simulink model "Main2016a"  (R2016a)
settings: Solver=ode45  StartTime=0.0  StopTime=t_end  FixedStep=st  MaxStep=st  RelTol=1e-3
values from neighbouring files (symbols this model uses):
  A = eye(16,16)    [full_input_list.m]
  counter = 0    [full_input_list.m]
  I_1 = [m*(zl^2+xyl^2)/12 0 0 ;          0 m*(zl^2+xyl^2)/12 0 ;          0 0 m*(2*xyl^2)/12 ] + 1e-6*(rand(3)-0.5)    [initACS.m]
  I_1_inv = inv(I_1)    [initACS.m]
  I_2 = [m*(zl^2+xyl^2)/12 0 0 ;          0 m*(zl^2+xyl^2)/12 0 ;          0 0 m*(2*xyl^2)/12 ] + 1e-6*(rand(3)-0.5)    [initACS.m]
  I_2_inv = inv(I_2)    [initACS.m]
  I_3 = [m*(zl^2+xyl^2)/12 0 0 ;          0 m*(zl^2+xyl^2)/12 0 ;          0 0 m*(2*xyl^2)/12 ] + 1e-6*(rand(3)-0.5)    [initACS.m]
  I_3_inv = inv(I_3)    [initACS.m]
  kd = 0.5    [full_input_list.m]    (also in initACS.m = 0.01)
  kp = 1    [full_input_list.m]    (also in initACS.m = 0.01)
  OpModes = [0 0 0]    [full_input_list.m]
  OpTimes = [0 1 2]    [full_input_list.m]
  SeperationTime = 30000    [full_input_list.m]
  state1_i = [ 0 0 0 , 0 0 0 , q4_0', w0_N]'    [full_input_list.m]
  state2_i = [ 0 0 (teth_length+side1Dim(1)/2+centerDim(3)/2+10*eps) , 0 -.1 0 ,      q4_0_Cube2' , w0_N ]'    [full_input_list.m]
  state3_i = [ 0 0 -(teth_length+side1Dim(1)/2+centerDim(3)/2+10*eps), 0 .1 0 ,      q4_0_Cube3' , w0_N ]'    [full_input_list.m]
  teth_k = teth_area*teth_modulus/teth_length    (= 33772.1210261)    [full_input_list.m]    (also in initACS.m = 10)
  teth_lo = 30    [full_input_list.m]    (also in initACS.m)
undefined symbols (not defined in the file or in its folder): DiscIntNeverNeededParam, Inertia, km, n, SolarDeployTime, solarpanel1_i, solarpanel2_i
libraries: SimMainLibrary x11, aerolibutil x10, simulink x1, vrlib x1, dspmathops x1
(part 1 of 2)
settings Model: Creator=dtk42  LastModifiedBy=cjtho
settings SolverCC: ZeroCrossAlgorithm=Adaptive
settings GRTTargetCC: GeneratePreprocessorConditionals=Use local settings

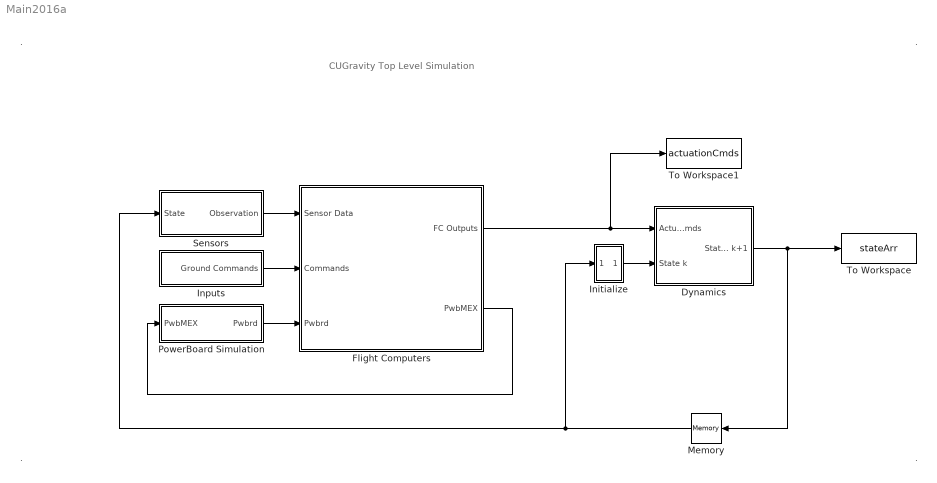
== system Main2016a ==
  note: .
  note: .
  note: .
  note: .
  note: CUGravity Top Level Simulation
  Dynamics : Subsystem
  Flight Computers : Subsystem
  Initialize : Subsystem
  Inputs : Subsystem
  Memory : Memory  InheritSampleTime=on
  PowerBoard Simulation : Subsystem
  Sensors : Subsystem
  To Workspace : ToWorkspace  VariableName=stateArr  SaveFormat=Timeseries  SampleTime=-1
  To Workspace1 : ToWorkspace  VariableName=actuationCmds  SaveFormat=Timeseries  SampleTime=-1
  wires:
  Sensors/1(Observation) -> Flight Computers/1(Sensor Data)
  Flight Computers/1(FC Outputs) -> Dynamics/1(Actuation Cmds), To Workspace1/1
  Initialize/1(xi) -> Dynamics/2(State k)
  Dynamics/1(State k+1) -> Memory/1, To Workspace/1
  Memory/1 -> Initialize/1(x), Sensors/1(State)
  Inputs/1(Ground Commands) -> Flight Computers/2(Commands)
  PowerBoard Simulation/1(Pwbrd) -> Flight Computers/3(Pwbrd)
  Flight Computers/2(PwbMEX) -> PowerBoard Simulation/1(PwbMEX)

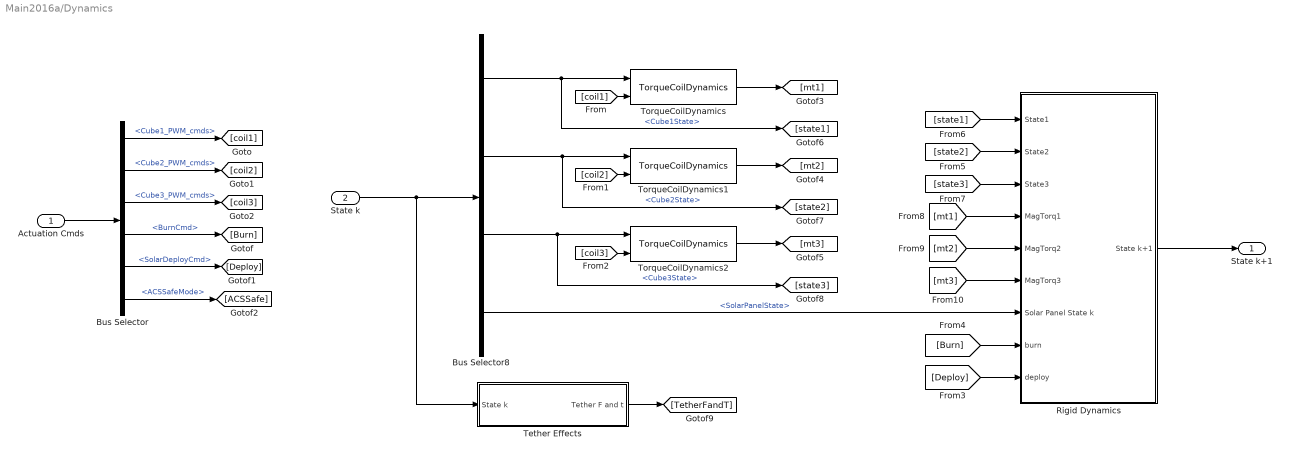
== system Main2016a/Dynamics ==
  Actuation Cmds : Inport
  State k : Inport  Port=2
  Bus Selector : BusSelector  OutputSignals=Cube1_PWM_cmds,Cube2_PWM_cmds,Cube3_PWM_cmds,BurnCmd,SolarDeployCmd,ACSSafeMode
  Bus Selector8 : BusSelector  OutputSignals=Cube1State,Cube2State,Cube3State,SolarPanelState
  Rigid Dynamics : Subsystem
  Tether Effects : Subsystem
  TorqueCoilDynamics : SimMainLibrary/TorqueCoilDynamics
  TorqueCoilDynamics1 : SimMainLibrary/TorqueCoilDynamics
  TorqueCoilDynamics2 : SimMainLibrary/TorqueCoilDynamics
  State k+1 : Outport
  wires:
  Bus Selector8/1 -> [state1], TorqueCoilDynamics/1  "<Cube1State>"
  Bus Selector8/2 -> TorqueCoilDynamics1/1, [state2]  "<Cube2State>"
  Bus Selector8/3 -> [state3], TorqueCoilDynamics2/1  "<Cube3State>"
  Bus Selector/1 -> [coil1]  "<Cube1_PWM_cmds>"
  Bus Selector/2 -> [coil2]  "<Cube2_PWM_cmds>"
  Bus Selector/3 -> [coil3]  "<Cube3_PWM_cmds>"
  [coil1] -> TorqueCoilDynamics/2
  [coil2] -> TorqueCoilDynamics1/2
  [coil3] -> TorqueCoilDynamics2/2
  Actuation Cmds/1 -> Bus Selector/1
  Bus Selector/4 -> [Burn]  "<BurnCmd>"
  Bus Selector/5 -> [Deploy]  "<SolarDeployCmd>"
  State k/1 -> Tether Effects/1(State k), Bus Selector8/1
  Rigid Dynamics/1(State k+1) -> State k+1/1
  Bus Selector/6 -> [ACSSafe]  "<ACSSafeMode>"
  TorqueCoilDynamics/1 -> [mt1]
  TorqueCoilDynamics1/1 -> [mt2]
  TorqueCoilDynamics2/1 -> [mt3]
  Tether Effects/1(Tether F and t) -> [TetherFandT]
  [Burn] -> Rigid Dynamics/8(burn)
  [Deploy] -> Rigid Dynamics/9(deploy)
  [state2] -> Rigid Dynamics/2(State2)
  [state1] -> Rigid Dynamics/1(State1)
  [state3] -> Rigid Dynamics/3(State3)
  [mt1] -> Rigid Dynamics/4(MagTorq1)
  [mt2] -> Rigid Dynamics/5(MagTorq2)
  [mt3] -> Rigid Dynamics/6(MagTorq3)
  Bus Selector8/4 -> Rigid Dynamics/7(Solar Panel State k)  "<SolarPanelState>"

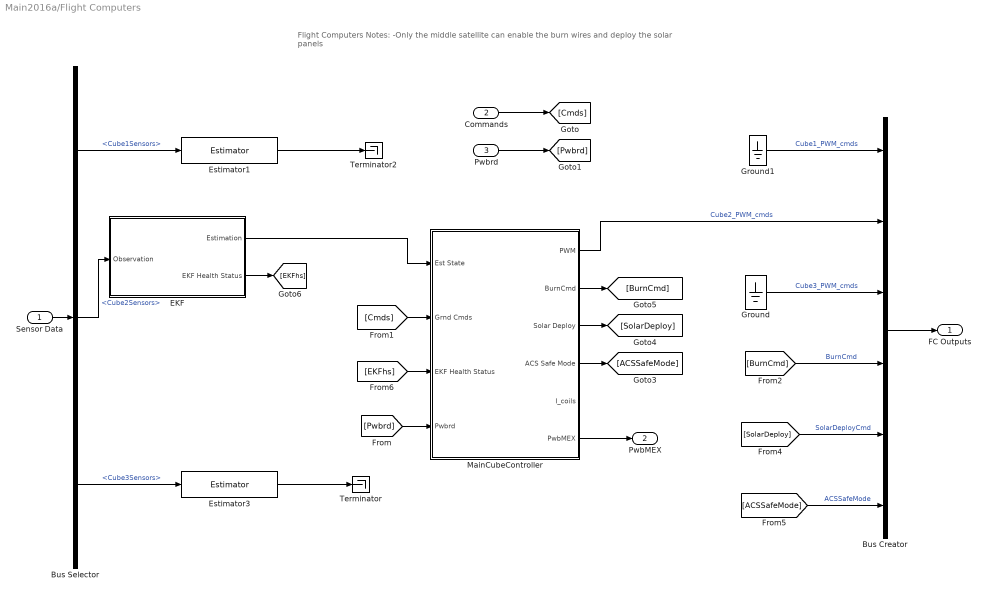
== system Main2016a/Flight Computers ==
  note: Flight Computers
      | Notes:
      | -Only the middle satellite can enable the burn wires and deploy the solar panels
  Sensor Data : Inport
  Commands : Inport  Port=2
  Pwbrd : Inport  Port=3
  Bus Creator : BusCreator  Inputs=6
  Bus Selector : BusSelector  OutputSignals=Cube1Sensors,Cube2Sensors,Cube3Sensors
  EKF : Subsystem  AncestorBlock=SimMainLibrary/Estimator
  Estimator1 : SimMainLibrary/Estimator
  Estimator3 : SimMainLibrary/Estimator
  Ground : Ground
  Ground1 : Ground
  MainCubeController : Subsystem  AncestorBlock=SimMainLibrary/MainCubeController
  Terminator : Terminator
  Terminator2 : Terminator
  FC Outputs : Outport
  PwbMEX : Outport  Port=2
  wires:
  Sensor Data/1 -> Bus Selector/1
  Bus Selector/1 -> Estimator1/1  "<Cube1Sensors>"
  EKF/1(Estimation) -> MainCubeController/1(Est State)
  Bus Selector/2 -> EKF/1(Observation)  "<Cube2Sensors>"
  MainCubeController/1(PWM) -> Bus Creator/2  "Cube2_PWM_cmds"
  Estimator3/1 -> Terminator/1
  Bus Selector/3 -> Estimator3/1  "<Cube3Sensors>"
  Estimator1/1 -> Terminator2/1
  Ground1/1 -> Bus Creator/1  "Cube1_PWM_cmds"
  Bus Creator/1 -> FC Outputs/1
  Ground/1 -> Bus Creator/3  "Cube3_PWM_cmds"
  Commands/1 -> [Cmds]
  [Cmds] -> MainCubeController/2(Grnd Cmds)
  MainCubeController/4(ACS Safe Mode) -> [ACSSafeMode]
  MainCubeController/3(Solar Deploy) -> [SolarDeploy]
  MainCubeController/2(BurnCmd) -> [BurnCmd]
  [BurnCmd] -> Bus Creator/4  "BurnCmd"
  [SolarDeploy] -> Bus Creator/5  "SolarDeployCmd"
  [ACSSafeMode] -> Bus Creator/6  "ACSSafeMode"
  EKF/2(EKF Health Status) -> [EKFhs]
  [EKFhs] -> MainCubeController/3("EKF Health Status ")
  Pwbrd/1 -> [Pwbrd]
  [Pwbrd] -> MainCubeController/4(Pwbrd)
  MainCubeController/6(PwbMEX) -> PwbMEX/1

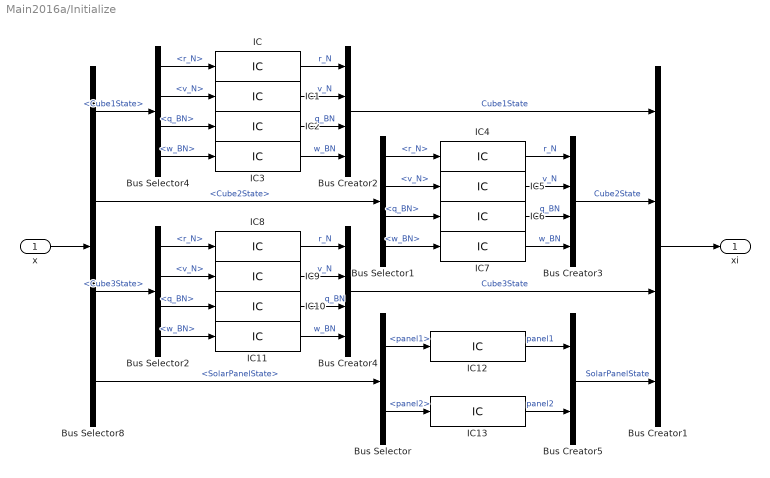
== system Main2016a/Initialize ==
  x : Inport
  Bus Creator1 : BusCreator  Inputs=4
  Bus Creator2 : BusCreator  Inputs='r_N','v_N','q_BN','w_BN'
  Bus Creator3 : BusCreator  Inputs='r_N','v_N','q_BN','w_BN'
  Bus Creator4 : BusCreator  Inputs='r_N','v_N','q_BN','w_BN'
  Bus Creator5 : BusCreator  Inputs='panel1','panel2'
  Bus Selector : BusSelector  OutputSignals=panel1,panel2
  Bus Selector1 : BusSelector  OutputSignals=r_N,v_N,q_BN,w_BN
  Bus Selector2 : BusSelector  OutputSignals=r_N,v_N,q_BN,w_BN
  Bus Selector4 : BusSelector  OutputSignals=r_N,v_N,q_BN,w_BN
  Bus Selector8 : BusSelector  OutputSignals=Cube1State,Cube2State,Cube3State,SolarPanelState
  IC : InitialCondition  Value=state1_i(1:3)
  IC1 : InitialCondition  Value=state1_i(4:6)
  IC10 : InitialCondition  Value=state3_i(7:10)
  IC11 : InitialCondition  Value=state3_i(11:13)
  IC12 : InitialCondition  Value=solarpanel1_i(1:4)
  IC13 : InitialCondition  Value=solarpanel2_i(1:4)
  IC2 : InitialCondition  Value=state1_i(7:10)
  IC3 : InitialCondition  Value=state1_i(11:13)
  IC4 : InitialCondition  Value=state2_i(1:3)
  IC5 : InitialCondition  Value=state2_i(4:6)
  IC6 : InitialCondition  Value=state2_i(7:10)
  IC7 : InitialCondition  Value=state2_i(11:13)
  IC8 : InitialCondition  Value=state3_i(1:3)
  IC9 : InitialCondition  Value=state3_i(4:6)
  xi : Outport
  wires:
  Bus Selector4/3 -> IC2/1  "<q_BN>"
  x/1 -> Bus Selector8/1
  Bus Creator1/1 -> xi/1
  Bus Selector8/1 -> Bus Selector4/1  "<Cube1State>"
  Bus Selector4/4 -> IC3/1  "<w_BN>"
  Bus Selector4/1 -> IC/1  "<r_N>"
  Bus Creator2/1 -> Bus Creator1/1  "Cube1State"
  Bus Selector4/2 -> IC1/1  "<v_N>"
  IC/1 -> Bus Creator2/1  "r_N"
  IC1/1 -> Bus Creator2/2  "v_N"
  IC2/1 -> Bus Creator2/3  "q_BN"
  IC3/1 -> Bus Creator2/4  "w_BN"
  Bus Selector1/3 -> IC6/1  "<q_BN>"
  Bus Selector1/4 -> IC7/1  "<w_BN>"
  Bus Selector1/1 -> IC4/1  "<r_N>"
  Bus Selector1/2 -> IC5/1  "<v_N>"
  Bus Selector8/2 -> Bus Selector1/1  "<Cube2State>"
  Bus Selector2/3 -> IC10/1  "<q_BN>"
  Bus Selector2/4 -> IC11/1  "<w_BN>"
  Bus Selector2/1 -> IC8/1  "<r_N>"
  Bus Selector2/2 -> IC9/1  "<v_N>"
  Bus Selector8/3 -> Bus Selector2/1  "<Cube3State>"
  IC4/1 -> Bus Creator3/1  "r_N"
  IC5/1 -> Bus Creator3/2  "v_N"
  IC6/1 -> Bus Creator3/3  "q_BN"
  IC7/1 -> Bus Creator3/4  "w_BN"
  Bus Creator4/1 -> Bus Creator1/3  "Cube3State"
  IC8/1 -> Bus Creator4/1  "r_N"
  IC9/1 -> Bus Creator4/2  "v_N"
  IC10/1 -> Bus Creator4/3  "q_BN"
  IC11/1 -> Bus Creator4/4  "w_BN"
  Bus Creator3/1 -> Bus Creator1/2  "Cube2State"
  Bus Selector8/4 -> Bus Selector/1  "<SolarPanelState>"
  Bus Creator5/1 -> Bus Creator1/4  "SolarPanelState"
  IC12/1 -> Bus Creator5/1  "panel1"
  IC13/1 -> Bus Creator5/2  "panel2"
  Bus Selector/1 -> IC12/1  "<panel1>"
  Bus Selector/2 -> IC13/1  "<panel2>"

== system Main2016a/Inputs ==
  Bus Creator : BusCreator  Inputs=3
  Choose Mode : MATLAB Function  TreatAsAtomicUnit=on
      settings: PermitHierarchicalResolution=ParametersOnly
  Clock : Clock
  Constant : Constant  Value=OpModes
  Constant1 : Constant  Value=OpTimes
  Constant2 : Constant  Value=SeperationTime
  Constant3 : Constant  Value=SolarDeployTime
  Ground Commands : Outport
  wires:
  Constant/1 -> Choose Mode/3(OpModes)
  Constant1/1 -> Choose Mode/2(OpTimes)
  Clock/1 -> Choose Mode/1(time)
  Constant2/1 -> Choose Mode/4(SeperationTime)
  Choose Mode/1(OM) -> Bus Creator/1  "OpMode"
  Choose Mode/2(SEPC) -> Bus Creator/2  "SeperationCommand"
  Bus Creator/1 -> Ground Commands/1
  Constant3/1 -> Choose Mode/5(SolarDeployTime)
  Choose Mode/3(SDC) -> Bus Creator/3  "SolarDeployCommand"

== system Main2016a/PowerBoard Simulation ==
  PwbMEX : Inport
  Bus Creator : BusCreator  Inputs=2
  Bus Creator1 : BusCreator  Inputs=8
  Bus Creator2 : BusCreator  Inputs=3
  Bus Creator3 : BusCreator  Inputs=2
  Bus Creator4 : BusCreator  Inputs=2
  Choose Mode : MATLAB Function  TreatAsAtomicUnit=on
      settings: PermitHierarchicalResolution=ParametersOnly
  Clock : Clock
  Constant : Constant  Value=OpModes
  Constant1 : Constant  Value=OpTimes
  Constant2 : Constant  Value=SeperationTime
  Constant3 : Constant  Value=SolarDeployTime
  Sensor Ak Signals : Subsystem
  Terminator : Terminator
  Torquer Shunts : Subsystem
  Pwbrd : Outport
  wires:
  Constant/1 -> Choose Mode/4(OpModes)
  Constant1/1 -> Choose Mode/3(OpTimes)
  Clock/1 -> Choose Mode/2(time)
  Constant2/1 -> Choose Mode/5(SeperationTime)
  Choose Mode/1(OM) -> Bus Creator/1  "PbOpMode"
  Choose Mode/2(SEPC) -> Bus Creator/2  "PbSepCmmd"
  Bus Creator/1 -> Bus Creator4/1  "PwbrdCmmds"
  Constant3/1 -> Choose Mode/6(SolarDeployTime)
  Choose Mode/3(SDC) -> Terminator/1  "SolarDeployCommand"
  Sensor Ak Signals/4(Out4) -> Bus Creator1/4  "Accel2Ak"
  Sensor Ak Signals/3(Out3) -> Bus Creator1/3  "Accel1Ak"
  Sensor Ak Signals/1(Out1) -> Bus Creator1/1  "Mag1Ak"
  Sensor Ak Signals/2(Out2) -> Bus Creator1/2  "Mag2Ak"
  Bus Creator1/1 -> Bus Creator3/1  "SensorsAk"
  Torquer Shunts/1(Torquer X1 Shunt) -> Bus Creator2/1  "TC_X1"
  Torquer Shunts/2(Torquer Y1 Shunt) -> Bus Creator2/2  "TC_Y1"
  Torquer Shunts/3(Torquer Z1 Shunt) -> Bus Creator2/3  "TC_Z1"
  Bus Creator2/1 -> Bus Creator3/2  "TorquerAk"
  Bus Creator3/1 -> Bus Creator4/2  "ADCSAks"
  Bus Creator4/1 -> Pwbrd/1
  Sensor Ak Signals/5(Out5) -> Bus Creator1/5  "Gyro1Ak"
  Sensor Ak Signals/6(Out6) -> Bus Creator1/6  "Gyro2Ak"
  Sensor Ak Signals/7(Out7) -> Bus Creator1/7  "SunS1Ak"
  Sensor Ak Signals/8(Out8) -> Bus Creator1/8  "SunS2Ak"
  PwbMEX/1 -> Choose Mode/1(PwbMEX)

== system Main2016a/Sensors ==
  State : Inport
  Bus Creator1 : BusCreator  Inputs=3
  Bus Selector1 : BusSelector  OutputSignals=Cube1State,Cube2State,Cube3State
  Rate Transition : RateTransition
  SensorsBlock1 : SimMainLibrary/SensorsBlock
  SensorsBlock2 : SimMainLibrary/SensorsBlock
  SensorsBlock3 : SimMainLibrary/SensorsBlock
  Observation : Outport
  wires:
  Bus Creator1/1 -> Observation/1
  State/1 -> Rate Transition/1
  Bus Selector1/1 -> SensorsBlock3/1  "<Cube1State>"
  SensorsBlock3/1 -> Bus Creator1/1  "Cube1Sensors"
  SensorsBlock2/1 -> Bus Creator1/3  "Cube3Sensors"
  SensorsBlock1/1 -> Bus Creator1/2  "Cube2Sensors"
  Bus Selector1/2 -> SensorsBlock1/1  "<Cube2State>"
  Bus Selector1/3 -> SensorsBlock2/1  "<Cube3State>"
  Rate Transition/1 -> Bus Selector1/1

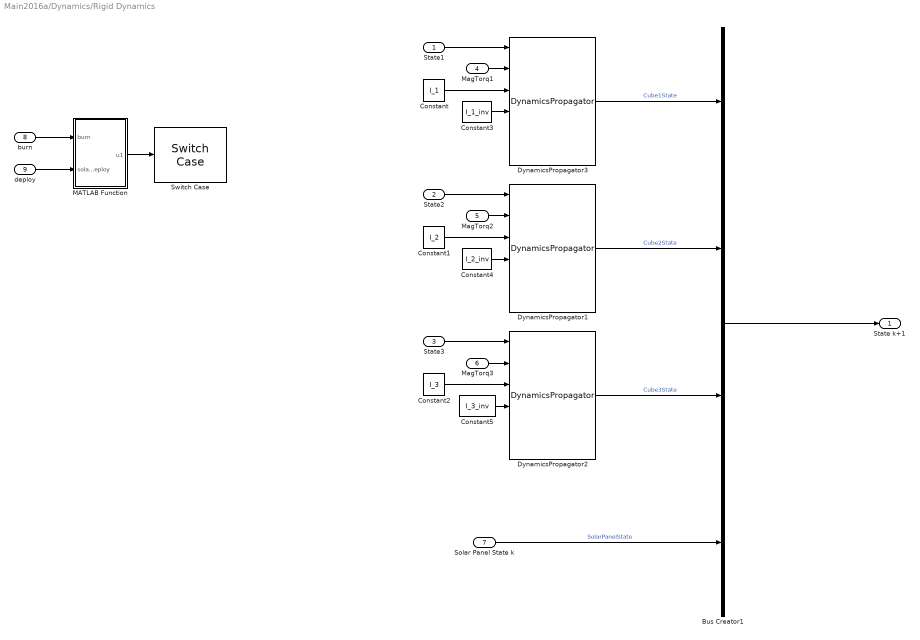
== system Main2016a/Dynamics/Rigid Dynamics ==
  State1 : Inport
  State2 : Inport  Port=2
  State3 : Inport  Port=3
  MagTorq1 : Inport  Port=4
  MagTorq2 : Inport  Port=5
  MagTorq3 : Inport  Port=6
  Solar Panel State k : Inport  Port=7
  burn : Inport  Port=8
  deploy : Inport  Port=9
  Bus Creator1 : BusCreator  Inputs='Cube1State','Cube2State','Cube3State','SolarPanelState'
  Constant : Constant  Value=I_1
  Constant1 : Constant  Value=I_2
  Constant2 : Constant  Value=I_3
  Constant3 : Constant  Value=I_1_inv
  Constant4 : Constant  Value=I_2_inv
  Constant5 : Constant  Value=I_3_inv
  DynamicsPropagator1 : SimMainLibrary/DynamicsPropagator
  DynamicsPropagator2 : SimMainLibrary/DynamicsPropagator
  DynamicsPropagator3 : SimMainLibrary/DynamicsPropagator
  MATLAB Function : MATLAB Function  TreatAsAtomicUnit=on
      settings: PermitHierarchicalResolution=ParametersOnly
  Switch Case : SwitchCase  CaseConditions={1,2,3}  ShowDefaultCase=off
  State k+1 : Outport
  wires:
  Constant2/1 -> DynamicsPropagator2/3
  Bus Creator1/1 -> State k+1/1
  DynamicsPropagator2/1 -> Bus Creator1/3  "Cube3State"
  Constant5/1 -> DynamicsPropagator2/4
  DynamicsPropagator1/1 -> Bus Creator1/2  "Cube2State"
  Constant4/1 -> DynamicsPropagator1/4
  Constant1/1 -> DynamicsPropagator1/3
  DynamicsPropagator3/1 -> Bus Creator1/1  "Cube1State"
  Constant3/1 -> DynamicsPropagator3/4
  Constant/1 -> DynamicsPropagator3/3
  State1/1 -> DynamicsPropagator3/1
  State2/1 -> DynamicsPropagator1/1
  State3/1 -> DynamicsPropagator2/1
  MagTorq1/1 -> DynamicsPropagator3/2
  MagTorq2/1 -> DynamicsPropagator1/2
  MagTorq3/1 -> DynamicsPropagator2/2
  Solar Panel State k/1 -> Bus Creator1/4  "SolarPanelState"
  MATLAB Function/1(u1) -> Switch Case/1
  burn/1 -> MATLAB Function/1(burn)
  deploy/1 -> MATLAB Function/2(solardeploy)

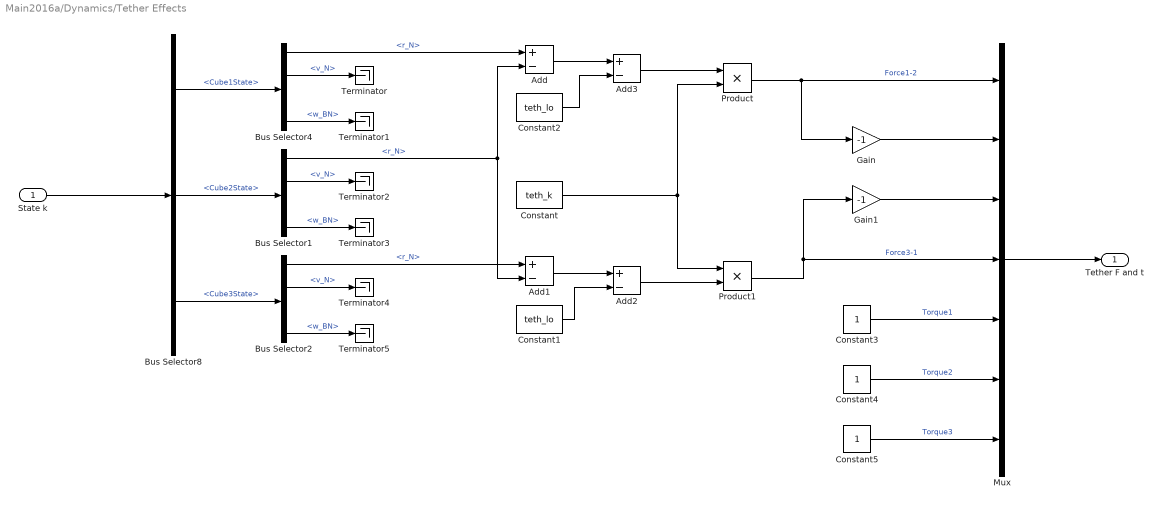
== system Main2016a/Dynamics/Tether Effects ==
  State k : Inport
  Add{,1..3} (4 alike) : Sum  Inputs=+-
  Bus Selector1 : BusSelector  OutputSignals=r_N,v_N,q_BN,w_BN
  Bus Selector2 : BusSelector  OutputSignals=r_N,v_N,q_BN,w_BN
  Bus Selector4 : BusSelector  OutputSignals=r_N,v_N,q_BN,w_BN
  Bus Selector8 : BusSelector  OutputSignals=Cube1State,Cube2State,Cube3State
  Constant : Constant  Value=teth_k
  Constant1 : Constant  Value=teth_lo
  Constant2 : Constant  Value=teth_lo
  Constant3 : Constant
  Constant4 : Constant
  Constant5 : Constant
  Gain : Gain  Gain=-1
  Gain1 : Gain  Gain=-1
  Mux : Mux  Inputs=7
  Product : Product
  Product1 : Product
  Terminator{,1..5} (6 alike) : Terminator
  Tether F and t : Outport
  wires:
  State k/1 -> Bus Selector8/1
  Bus Selector8/1 -> Bus Selector4/1  "<Cube1State>"
  Bus Selector8/2 -> Bus Selector1/1  "<Cube2State>"
  Bus Selector8/3 -> Bus Selector2/1  "<Cube3State>"
  Bus Selector4/2 -> Terminator/1  "<v_N>"
  Bus Selector4/4 -> Terminator1/1  "<w_BN>"
  Bus Selector1/2 -> Terminator2/1  "<v_N>"
  Bus Selector1/4 -> Terminator3/1  "<w_BN>"
  Bus Selector2/2 -> Terminator4/1  "<v_N>"
  Bus Selector2/4 -> Terminator5/1  "<w_BN>"
  Bus Selector4/1 -> Add/1  "<r_N>"
  Bus Selector1/1 -> Add1/2, Add/2  "<r_N>"
  Bus Selector2/1 -> Add1/1  "<r_N>"
  Add/1 -> Add3/1
  Constant/1 -> Product1/1, Product/2
  Add1/1 -> Add2/1
  Product/1 -> Gain/1, Mux/1  "Force1-2"
  Product1/1 -> Gain1/1, Mux/4  "Force3-1"
  Add2/1 -> Product1/2
  Constant1/1 -> Add2/2
  Constant2/1 -> Add3/2
  Add3/1 -> Product/1
  Constant3/1 -> Mux/5  "Torque1"
  Gain/1 -> Mux/2
  Gain1/1 -> Mux/3
  Constant4/1 -> Mux/6  "Torque2"
  Constant5/1 -> Mux/7  "Torque3"
  Mux/1 -> Tether F and t/1

== system Main2016a/Flight Computers/EKF ==
  note: This is the Kalman filter. The goal of the Kalman filter is to obtain an estimate of the craft's attitude based off of sensor data from the previous state. it does so by taking in sensor data, creating an estimate of the attitude from said data, saving it, and comparing the next state iteration with its estimate in order to determine the accuracy and the validity of each component of the sensor data.
  note: Kalman Filter
  note: The output of this block should be both an estimate of the attitude based off of the sensor data (as well as historical values), as well as a boolean value for the EKF Health Status determined by the covariance matrix.
  Observation : Inport
  Add : Sum
  Average : Product  Inputs=*/
  Bus Creator : BusCreator  Inputs=4
  Bus Selector : BusSelector  OutputSignals=r_N,a_N,q_BN,w_BN
  Constant : Constant  Value=2
  Constant1 : Constant
  Discrete Derivative : simulink/Discrete/Discrete Derivative  gainval=1.0  ICPrevScaledInput=0.0  OutMin=[]  OutMax=[]  OutDataType=fixdt(1, 16)  OutScaling=2^-10  DoSatur=off
  Discrete Filter : DiscreteFilter
  Discrete Filter1 : DiscreteFilter
  Discrete Filter2 : DiscreteFilter
  Discrete-Time Integrator : DiscreteIntegrator  InitialConditionSetting=State (most efficient)  SampleTime=-1  ICPrevOutput=DiscIntNeverNeededParam  ICPrevScaledInput=DiscIntNeverNeededParam
  Estimation : Outport
  EKF Health Status : Outport  Port=2
  wires:
  Bus Selector/2 -> Discrete-Time Integrator/1  "<a_N>"
  Discrete-Time Integrator/1 -> Add/2
  Discrete Derivative/1 -> Add/1
  Discrete Filter/1 -> Bus Creator/1  "r_N_est"
  Bus Selector/4 -> Discrete Filter2/1  "<w_BN>"
  Add/1 -> Average/1
  Constant/1 -> Average/2
  Average/1 -> Bus Creator/2  "v_N_est"
  Bus Selector/1 -> Discrete Derivative/1, Discrete Filter/1  "<r_N>"
  Bus Selector/3 -> Discrete Filter1/1  "<q_BN>"
  Observation/1 -> Bus Selector/1
  Bus Creator/1 -> Estimation/1
  Discrete Filter2/1 -> Bus Creator/4  "w_BN_est"
  Discrete Filter1/1 -> Bus Creator/3  "q_BN_est"
  Constant1/1 -> EKF Health Status/1

== system Main2016a/Flight Computers/MainCubeController ==
  note: Work Notes
      |
      | I am starting to work on the estimator
  Est State : Inport
  Grnd Cmds : Inport  Port=2
  "EKF Health Status " : Inport  Port=3
  Pwbrd : Inport  Port=4
  GNC : Subsystem
  Memory : Memory  InheritSampleTime=on
  Navigation : Subsystem
  SafeMode : Subsystem
  Terminator2 : Terminator
  Terminator3 : Terminator
  PWM : Outport
  BurnCmd : Outport  Port=2
  Solar Deploy : Outport  Port=3
  ACS Safe Mode : Outport  Port=4
  I_coils : Outport  Port=5
  PwbMEX : Outport  Port=6
  wires:
  Memory/1 -> SafeMode/3(Safe Mode In)
  GNC/1(OpMode) -> Navigation/1(BurnCmd)
  GNC/3(SolarDeploy) -> Solar Deploy/1
  GNC/2(SepBurn) -> BurnCmd/1
  SafeMode/3(SafedSolarDeploy) -> GNC/3(SafedSolarDeploy)
  SafeMode/2(SafedSeperationBurn) -> GNC/2(SafedSepBurn)
  SafeMode/4(SafedPos) -> Terminator3/1
  SafeMode/5(SafedVel) -> Terminator2/1
  Est State/1 -> SafeMode/2(EstState)
  SafeMode/1(SafedOpMode) -> GNC/1(SafedOpMode)
  Grnd Cmds/1 -> SafeMode/1(GrndCmds)
  "EKF Health Status "/1 -> SafeMode/5("EKFhs ")
  Pwbrd/1 -> SafeMode/4(Pwbrd)
  Navigation/2(torque_coils) -> PWM/1
  Navigation/1(current_coils) -> I_coils/1
  GNC/4(Tau1) -> Navigation/4(tau_B)
  SafeMode/6(Safed q) -> Navigation/2(q_BN), GNC/4(q2)
  SafeMode/8(Safe Mode Out) -> Memory/1, ACS Safe Mode/1
  SafeMode/9(PwbMEX) -> PwbMEX/1
  SafeMode/7(Safed w) -> Navigation/3(w), GNC/5(w2)

== system Main2016a/PowerBoard Simulation/Sensor Ak Signals ==
  Acc1 : Constant
  Acc2 : Constant
  Gyro1 : Constant
  Gyro2 : Constant
  Mag1 : Constant
  Mag2 : Constant
  SunSensor1 : Constant
  SunSensor2 : Constant
  Out1 : Outport
  Out2 : Outport  Port=2
  Out3 : Outport  Port=3
  Out4 : Outport  Port=4
  Out5 : Outport  Port=5
  Out6 : Outport  Port=6
  Out7 : Outport  Port=7
  Out8 : Outport  Port=8
  wires:
  Acc2/1 -> Out4/1
  Acc1/1 -> Out3/1
  Mag2/1 -> Out2/1
  Mag1/1 -> Out1/1
  Gyro2/1 -> Out6/1
  Gyro1/1 -> Out5/1
  SunSensor1/1 -> Out7/1
  SunSensor2/1 -> Out8/1

== system Main2016a/PowerBoard Simulation/Torquer Shunts ==
  Constant : Constant
  Constant2 : Constant
  Constant4 : Constant
  Torquer X1 Shunt : Outport
  Torquer Y1 Shunt : Outport  Port=2
  Torquer Z1 Shunt : Outport  Port=3
  wires:
  Constant4/1 -> Torquer Z1 Shunt/1
  Constant2/1 -> Torquer Y1 Shunt/1
  Constant/1 -> Torquer X1 Shunt/1

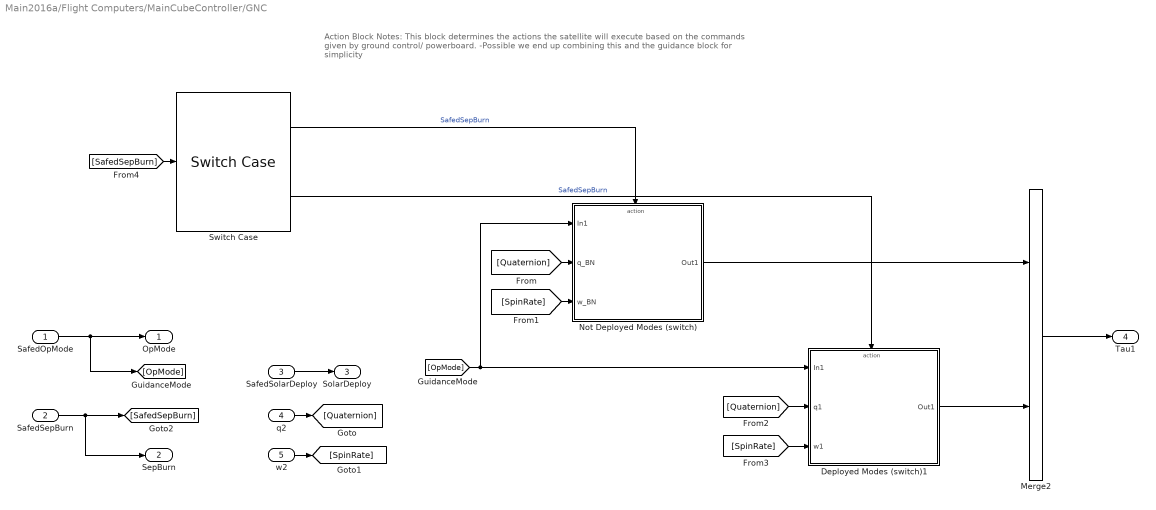
== system Main2016a/Flight Computers/MainCubeController/GNC ==
  note: Action Block
      | Notes: This block determines the actions the satellite will execute based on the commands given by ground control/ powerboard.
      | -Possible we end up combining this and the guidance block for simplicity
  SafedOpMode : Inport
  SafedSepBurn : Inport  Port=2
  SafedSolarDeploy : Inport  Port=3
  q2 : Inport  Port=4
  w2 : Inport  Port=5
  Deployed Modes (switch)1 : Subsystem
  Merge2 : Merge
  Not Deployed Modes (switch) : Subsystem
  Switch Case : SwitchCase  CaseConditions={0,1}  ShowDefaultCase=off
  OpMode : Outport
  SepBurn : Outport  Port=2
  SolarDeploy : Outport  Port=3
  Tau1 : Outport  Port=4
  wires:
  SafedOpMode/1 -> [OpMode], OpMode/1
  SafedSolarDeploy/1 -> SolarDeploy/1
  Merge2/1 -> Tau1/1
  Not Deployed Modes (switch)/1(Out1) -> Merge2/1
  q2/1 -> [Quaternion]
  w2/1 -> [SpinRate]
  [Quaternion] -> Not Deployed Modes (switch)/2(q_BN)
  [SpinRate] -> Not Deployed Modes (switch)/3(w_BN)
  [Quaternion] -> Deployed Modes (switch)1/2(q1)
  [SpinRate] -> Deployed Modes (switch)1/3(w1)
  Deployed Modes (switch)1/1(Out1) -> Merge2/2
  [SafedSepBurn] -> Switch Case/1
  SafedSepBurn/1 -> SepBurn/1, [SafedSepBurn]
  Switch Case/1 -> Not Deployed Modes (switch)/Action  "SafedSepBurn"
  Switch Case/2 -> Deployed Modes (switch)1/Action  "SafedSepBurn"
  [OpMode] -> Deployed Modes (switch)1/1(In1), Not Deployed Modes (switch)/1(In1)

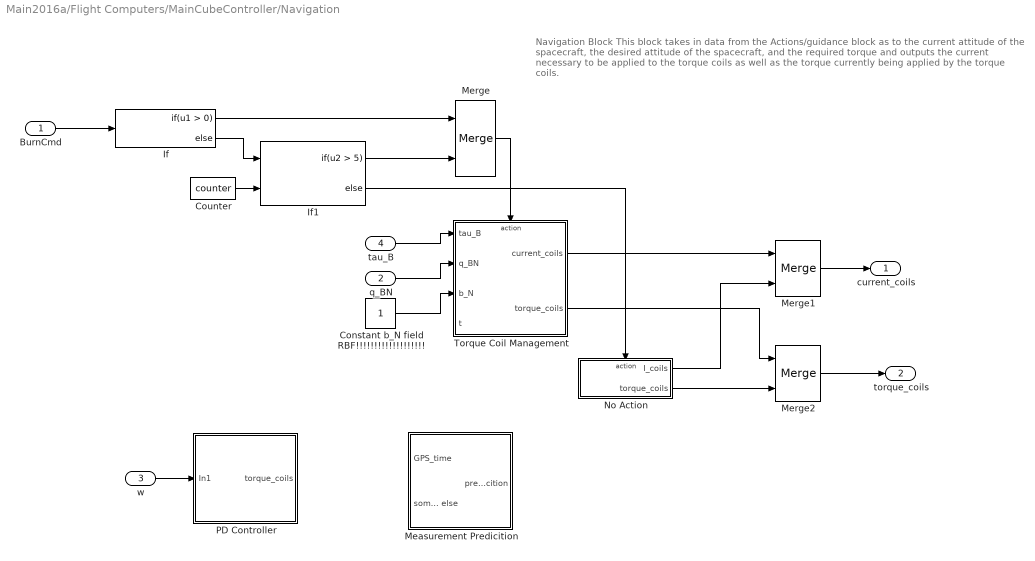
== system Main2016a/Flight Computers/MainCubeController/Navigation ==
  note: Navigation Block
      | This block takes in data from the Actions/guidance block as to the current attitude of the spacecraft, the desired attitude of the spacecraft, and the required torque and outputs the current necessary to be applied to the torque coils as well as the torque currently being applied by the torque coils.
  BurnCmd : Inport
  q_BN : Inport  Port=2
  w : Inport  Port=3
  tau_B : Inport  Port=4
  Constant b_N field RBF!!!!!!!!!!!!!!!!!!! : Constant
  Counter : Constant  Value=counter
  If : If
  If1 : If  NumInputs=2  IfExpression=u2 > 5
  Measurement Predicition : Subsystem
  Merge : Merge
  Merge1 : Merge
  Merge2 : Merge
  No Action : Subsystem  TreatAsAtomicUnit=on
  PD Controller : Subsystem
  Torque Coil Management : Subsystem  TreatAsAtomicUnit=on
  current_coils : Outport
  torque_coils : Outport  Port=2
  wires:
  Constant b_N field RBF!!!!!!!!!!!!!!!!!!!/1 -> Torque Coil Management/3(b_N)
  BurnCmd/1 -> If/1
  If/2 -> If1/1
  If/1 -> Merge/1
  If1/1 -> Merge/2
  Merge/1 -> Torque Coil Management/Action
  Merge1/1 -> current_coils/1
  Merge2/1 -> torque_coils/1
  If1/2 -> No Action/Action
  Torque Coil Management/1(current_coils) -> Merge1/1
  Torque Coil Management/2(torque_coils) -> Merge2/1
  No Action/1(I_coils) -> Merge1/2
  No Action/2(torque_coils) -> Merge2/2
  Counter/1 -> If1/2
  q_BN/1 -> Torque Coil Management/2(q_BN)
  tau_B/1 -> Torque Coil Management/1(tau_B)
  w/1 -> PD Controller/1(In1)

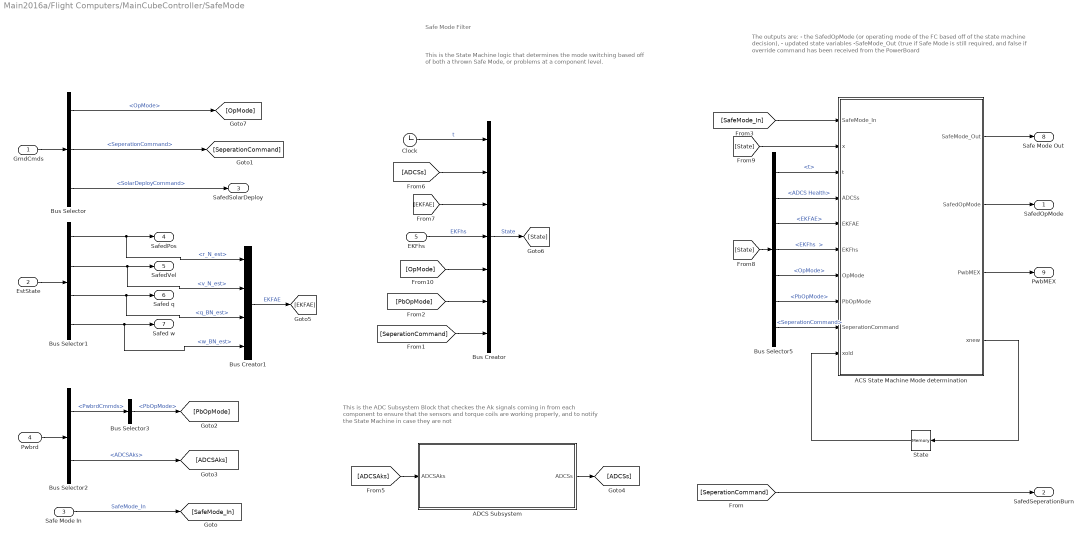
== system Main2016a/Flight Computers/MainCubeController/SafeMode ==
  note: This is the State Machine logic that determines the mode switching based off of both a thrown Safe Mode, or problems at a component level.
  note: Safe Mode Filter
  note: The outputs are:
      | - the SafedOpMode (or operating mode of the FC based off of the state machine decision),
      | - updated state variables
      | -SafeMode_Out (true if Safe Mode is still required, and false if override command has been received from the PowerBoard
  note: This is the ADC Subsystem Block that checkes the Ak signals coming in from each component to ensure that the sensors and torque coils are working properly, and to notify the State Machine in case they are not
  GrndCmds : Inport
  EstState : Inport  Port=2
  Safe Mode In : Inport  Port=3
  Pwbrd : Inport  Port=4
  "EKFhs " : Inport  Port=5
  ACS State Machine Mode determination : MATLAB Function  TreatAsAtomicUnit=on
      settings: PermitHierarchicalResolution=ParametersOnly
  ADCS Subsystem : Subsystem
  Bus Creator : BusCreator  Inputs=7
  Bus Creator1 : BusCreator  Inputs=4
  Bus Selector : BusSelector  OutputSignals=OpMode,SeperationCommand,SolarDeployCommand
  Bus Selector1 : BusSelector  OutputSignals=r_N_est,v_N_est,q_BN_est,w_BN_est
  Bus Selector2 : BusSelector  OutputSignals=PwbrdCmmds,ADCSAks
  Bus Selector3 : BusSelector  OutputSignals=PbOpMode
  Bus Selector5 : BusSelector  OutputSignals="t,ADCS Health,EKFAE,EKFhs  ,OpMode,PbOpMode,SeperationCommand"
  Clock : Clock
  State : Memory
  SafedOpMode : Outport
  SafedSeperationBurn : Outport  Port=2
  SafedSolarDeploy : Outport  Port=3
  SafedPos : Outport  Port=4
  SafedVel : Outport  Port=5
  Safed q : Outport  Port=6
  Safed w : Outport  Port=7
  Safe Mode Out : Outport  Port=8
  PwbMEX : Outport  Port=9
  wires:
  Clock/1 -> Bus Creator/1  "t"
  "EKFhs "/1 -> Bus Creator/4  "EKFhs"
  [ADCSs] -> Bus Creator/2
  Bus Selector1/4 -> Bus Creator1/4, Safed w/1  "<w_BN_est>"
  Bus Selector1/3 -> Bus Creator1/3, Safed q/1  "<q_BN_est>"
  Bus Selector1/2 -> Bus Creator1/2, SafedVel/1  "<v_N_est>"
  Bus Selector1/1 -> Bus Creator1/1, SafedPos/1  "<r_N_est>"
  EstState/1 -> Bus Selector1/1
  Bus Selector/3 -> SafedSolarDeploy/1  "<SolarDeployCommand>"
  Bus Selector/1 -> [OpMode]  "<OpMode>"
  GrndCmds/1 -> Bus Selector/1
  Safe Mode In/1 -> [SafeMode_In]  "SafeMode_In"
  ACS State Machine Mode determination/1(SafeMode_Out) -> Safe Mode Out/1
  Bus Selector/2 -> [SeperationCommand]  "<SeperationCommand>"
  [SeperationCommand] -> SafedSeperationBurn/1
  [SeperationCommand] -> Bus Creator/7
  State/1 -> ACS State Machine Mode determination/10(xold)
  Pwbrd/1 -> Bus Selector2/1
  Bus Selector2/2 -> [ADCSAks]  "<ADCSAks>"
  [ADCSAks] -> ADCS Subsystem/1("ADCSAks ")
  ADCS Subsystem/1("ADCSs ") -> [ADCSs]
  Bus Selector2/1 -> Bus Selector3/1  "<PwbrdCmmds>"
  Bus Selector3/1 -> [PbOpMode]  "<PbOpMode>"
  [SafeMode_In] -> ACS State Machine Mode determination/1(SafeMode_In)
  [OpMode] -> Bus Creator/5
  [PbOpMode] -> Bus Creator/6
  Bus Selector5/7 -> ACS State Machine Mode determination/9(SeperationCommand)  "<SeperationCommand>"
  Bus Selector5/6 -> ACS State Machine Mode determination/8(PbOpMode)  "<PbOpMode>"
  Bus Selector5/5 -> ACS State Machine Mode determination/7(OpMode)  "<OpMode>"
  Bus Selector5/4 -> ACS State Machine Mode determination/6(EKFhs)  "<EKFhs  >"
  Bus Selector5/3 -> ACS State Machine Mode determination/5(EKFAE)  "<EKFAE>"
  Bus Selector5/2 -> ACS State Machine Mode determination/4(ADCSs)  "<ADCS Health>"
  Bus Selector5/1 -> ACS State Machine Mode determination/3(t)  "<t>"
  Bus Creator1/1 -> [EKFAE]  "EKFAE"
  [EKFAE] -> Bus Creator/3
  Bus Creator/1 -> [State]  "State"
  [State] -> Bus Selector5/1
  [State] -> ACS State Machine Mode determination/2(x)
  ACS State Machine Mode determination/2(SafedOpMode) -> SafedOpMode/1
  ACS State Machine Mode determination/4(xnew) -> State/1
  ACS State Machine Mode determination/3(PwbMEX) -> PwbMEX/1

== system Main2016a/Flight Computers/MainCubeController/GNC/Deployed Modes (switch)1 ==
  note: Deployed Block
      | Notes: This block determines the actions the satellite will execute based on the commands given by ground control/ powerboard. The 2 cases are normal operations, and eclipse
  In1 : Inport
  q1 : Inport  Port=2
  w1 : Inport  Port=3
  Action Port : ActionPort  ActionType=case
  Bus Selector : BusSelector  OutputSignals=mode,SafedSepBurn
  Default : Subsystem  TreatAsAtomicUnit=on
  Deployed : SwitchCase  CaseConditions={7, 12}
  Merge1 : Merge  Inputs=3
  Seek EKF Convergence : Subsystem  TreatAsAtomicUnit=on
  Spin-Up Slew : Subsystem  TreatAsAtomicUnit=on
  Terminator : Terminator
  Out1 : Outport
  wires:
  w1/1 -> Spin-Up Slew/2(w)
  Deployed/1 -> Spin-Up Slew/Action
  Spin-Up Slew/1(tau) -> Merge1/1
  q1/1 -> Spin-Up Slew/1(q)
  Deployed/3 -> Default/Action
  Merge1/1 -> Out1/1
  In1/1 -> Bus Selector/1
  Bus Selector/1 -> Deployed/1  "<mode>"
  Bus Selector/2 -> Terminator/1  "<SafedSepBurn>"
  Default/1(Out1) -> Merge1/3
  Deployed/2 -> Seek EKF Convergence/Action
  Seek EKF Convergence/1(Out1) -> Merge1/2

== system Main2016a/Flight Computers/MainCubeController/GNC/Not Deployed Modes (switch) ==
  note: Not Deployed Block
      | Notes: This block determines the actions the satellite will execute based on the commands given by ground control/ powerboard. The 3 cases are detumbling, sun pointing, and eclipse
  In1 : Inport
  q_BN : Inport  Port=2
  w_BN : Inport  Port=3
  Action Port : ActionPort  ActionType=case
  Bus Selector : BusSelector  OutputSignals=SafedSepBurn,mode
  Detumbling Slew : Subsystem  TreatAsAtomicUnit=on
  Inertia : Constant  Value=Inertia
  Inital Spin Up : Subsystem  TreatAsAtomicUnit=on
  Merge1 : Merge  Inputs=5
  Not Deployed : SwitchCase  CaseConditions={5,6,7,12}
  Null Case1 : Subsystem  TreatAsAtomicUnit=on
  Seek EKF Convergence : Subsystem  TreatAsAtomicUnit=on
  Sun Pointing : Subsystem  TreatAsAtomicUnit=on
  Terminator : Terminator
  Out1 : Outport
  wires:
  Merge1/1 -> Out1/1
  Not Deployed/5 -> Null Case1/Action
  q_BN/1 -> Sun Pointing/1(q), Inital Spin Up/1(q_BN), Detumbling Slew/1(q_BN)
  Detumbling Slew/1(tau) -> Merge1/1
  Not Deployed/2 -> Sun Pointing/Action
  Sun Pointing/1(tau) -> Merge1/2
  Not Deployed/1 -> Detumbling Slew/Action
  w_BN/1 -> Detumbling Slew/2(w_BN), Sun Pointing/2(w_BN), Inital Spin Up/2(w)
  In1/1 -> Bus Selector/1
  Bus Selector/2 -> Not Deployed/1  "<mode>"
  Bus Selector/1 -> Terminator/1  "<SafedSepBurn>"
  Not Deployed/3 -> Inital Spin Up/Action
  Inital Spin Up/1(tau) -> Merge1/3
  Inertia/1 -> Inital Spin Up/3("I "), Detumbling Slew/3("I ")
  Not Deployed/4 -> Seek EKF Convergence/Action
  Null Case1/1(Out1) -> Merge1/5
  Seek EKF Convergence/1(Out1) -> Merge1/4

== system Main2016a/Flight Computers/MainCubeController/Navigation/Measurement Predicition ==
  note: Predicitoon Block
      | This block takes in the current time and the expected time when the action will be executed in order to give a better predicition of what the attitude of the satellite will be at.
  GPS_time : Inport
  something else : Inport  Port=2
  predicition : Outport

== system Main2016a/Flight Computers/MainCubeController/Navigation/No Action ==
  Action Port : ActionPort
  Constant : Constant  Value=[ 0 0 0 ]
  Constant2 : Constant  Value=[ 0 0 0 ]
  I_coils : Outport
  torque_coils : Outport  Port=2
  wires:
  Constant/1 -> I_coils/1
  Constant2/1 -> torque_coils/1

== system Main2016a/Flight Computers/MainCubeController/Navigation/PD Controller ==
  note: Controller
      | At this moment in time, I am not sure what this block does, but it appears to be a PD controller with feedforward control that outputs the torque the coils are required to exert. In short, a simple/not-simple controller
  In1 : Inport
  torque_coils : Outport

== system Main2016a/Flight Computers/MainCubeController/Navigation/Torque Coil Management ==
  tau_B : Inport
  q_BN : Inport  Port=2
  b_N : Inport  Port=3
  t : Inport  Port=4
  Action Port : ActionPort
  B_Q_N : MATLAB Function  TreatAsAtomicUnit=on
      settings: PermitHierarchicalResolution=ParametersOnly
  Cross Product : vrlib/Utilities/Cross Product
  Gain : Gain  Gain=km/(n*A)
  Gain1 : Gain  Gain=n*A
  I_PWMOutput Function : MATLAB Function  TreatAsAtomicUnit=on
      settings: PermitHierarchicalResolution=ParametersOnly
  Normalization : dspmathops/Normalization  NormType=Squared 2-norm  Bias=1e-10  NormOver=Each column  Dimension=1  outputDataTypeStr=Inherit: Same as product output  outputLastDataTypeStr=Inherit: Same as product output  outputMin=[]  outputMax=[]  accumDataTypeStr=Inherit: Same as product output  accumLastDataTypeStr=Inherit: Same as product output  roundingMode=Floor  overflowMode=off
  Product : Product  Multiplication=Matrix(*)
  current_coils : Outport
  torque_coils : Outport  Port=2
  wires:
  B_Q_N/1(DCM) -> Product/1
  q_BN/1 -> B_Q_N/1(q_BN)
  b_N/1 -> Product/2
  Product/1 -> Normalization/1
  Normalization/1 -> Cross Product/2
  tau_B/1 -> Cross Product/1
  I_PWMOutput Function/1(pwm) -> current_coils/1, Gain1/1
  Cross Product/1 -> Gain/1
  Gain/1 -> I_PWMOutput Function/1(I_des)
  Gain1/1 -> torque_coils/1
  t/1 -> I_PWMOutput Function/2(t)

== system Main2016a/Flight Computers/MainCubeController/SafeMode/ADCS Subsystem ==
  "ADCSAks " : Inport
  Bus Selector : BusSelector  OutputSignals=SensorsAk,TorquerAk
  Bus Selector1 : BusSelector  OutputSignals=Mag1Ak,Mag2Ak,Accel1Ak,Accel2Ak,Gyro1Ak,Gyro2Ak,SunS1Ak,SunS2Ak
  Bus Selector2 : BusSelector  OutputSignals=TC_X1,TC_Y1,TC_Z1
  IMU : Subsystem
  Logical Operator1 : Logic  Operator=OR  AllPortsSameDT=off  OutDataTypeStr=boolean
  Magnetic Torquers : Subsystem
  Mux : Mux
  Mux1 : Mux  Inputs=3
  Mux3 : Mux  Inputs=3
  Mux4 : Mux  Inputs=2
  Mux5 : Mux  Inputs=2
  "ADCSs " : Outport
  wires:
  Bus Selector2/3 -> Magnetic Torquers/3(Magnetometer Z1)  "<TC_Z1>"
  Bus Selector2/2 -> Magnetic Torquers/2(Magnetometer Y1)  "<TC_Y1>"
  Mux1/1 -> "ADCSs "/1  "ADCS Health"
  Mux4/1 -> Mux1/2  "ADCS Sectional Status"
  IMU/1(Magnetometer) -> Mux/1  "Magnetometer Health"
  IMU/3(Accelerometer) -> Mux/3  "Accelerometer Health"
  IMU/2("Gyro ") -> Mux/2  "Gyro Health"
  IMU/5(IMU Health) -> Mux4/1, Logical Operator1/1  "IMU Health"
  Magnetic Torquers/2("Y Torquer Status ") -> Mux3/2  "Y Torquer Status"
  Magnetic Torquers/1(X Torquer Status) -> Mux3/1  "X Torquer Status"
  Bus Selector2/1 -> Magnetic Torquers/1(Magnetorquer X1)  "<TC_X1>"
  IMU/4("Sun Sensor ") -> Mux/4  "Sun Sensor"
  Logical Operator1/1 -> Mux1/1  "ADCS Functional Status"
  Mux5/1 -> Mux1/3  "ADCS Component Status"
  Mux3/1 -> Mux5/2  "Torquer Status Array"
  Magnetic Torquers/4(Actuator Health) -> Mux4/2, Logical Operator1/2  "Actuator Health"
  Mux/1 -> Mux5/1  "Sensor Status Array"
  Magnetic Torquers/3(Z Torquer Status) -> Mux3/3  "Z Torquer Status"
  "ADCSAks "/1 -> Bus Selector/1
  Bus Selector/2 -> Bus Selector2/1  "<TorquerAk>"
  Bus Selector/1 -> Bus Selector1/1  "<SensorsAk>"
  Bus Selector1/1 -> IMU/1(Magnetometer 1)  "<Mag1Ak>"
  Bus Selector1/2 -> IMU/2(Magnetometer 2)  "<Mag2Ak>"
  Bus Selector1/3 -> IMU/3(Accelerometer 1)  "<Accel1Ak>"
  Bus Selector1/4 -> IMU/4(" Accelerometer 2")  "<Accel2Ak>"
  Bus Selector1/5 -> IMU/5(Gyro 1)  "<Gyro1Ak>"
  Bus Selector1/6 -> IMU/6(Gyro 2)  "<Gyro2Ak>"
  Bus Selector1/7 -> IMU/7(Sun Sensor 1)  "<SunS1Ak>"
  Bus Selector1/8 -> IMU/8(Sun Sensor 2)  "<SunS2Ak>"

== system Main2016a/Flight Computers/MainCubeController/GNC/Deployed Modes (switch)1/Default ==
  Action Port : ActionPort
  Constant : Constant  Value=[ 0 0 0 ]
  Out1 : Outport
  wires:
  Constant/1 -> Out1/1

== system Main2016a/Flight Computers/MainCubeController/GNC/Deployed Modes (switch)1/Seek EKF Convergence ==
  Action Port : ActionPort  ActionType=case
  Constant : Constant  Value=[ 0 0 0 ]
  Out1 : Outport
  wires:
  Constant/1 -> Out1/1

== system Main2016a/Flight Computers/MainCubeController/GNC/Deployed Modes (switch)1/Spin-Up Slew ==
  note: Regulator
      | - q_target = [0 0 0 1]
      | - w_target = [0 0 0]
  q : Inport
  w : Inport  Port=2
  Action Port : ActionPort
  Add : Sum
  Gain : Gain  Gain=-1
  Gain1 : Gain  Gain=kp
  Gain2 : Gain  Gain=-1
  Gain3 : Gain  Gain=kd
  Quaternion Inverse : aerolibutil/Quaternion Inverse
  Quaternion Multiplication : aerolibutil/Quaternion Multiplication
  Selector : Selector  InputPortWidth=4  IndexOptions=Index vector (dialog)  Indices=[1 2 3]  OutputSizes=1
  Target q : Constant  Value=[ 0 0 0 1 ]
  tau : Outport
  wires:
  Gain2/1 -> Add/2
  Gain/1 -> Add/1
  Add/1 -> tau/1
  w/1 -> Gain3/1
  Gain3/1 -> Gain2/1
  Gain1/1 -> Gain/1
  Selector/1 -> Gain1/1
  Quaternion Multiplication/1 -> Selector/1
  Target q/1 -> Quaternion Inverse/1
  Quaternion Inverse/1 -> Quaternion Multiplication/2
  q/1 -> Quaternion Multiplication/1

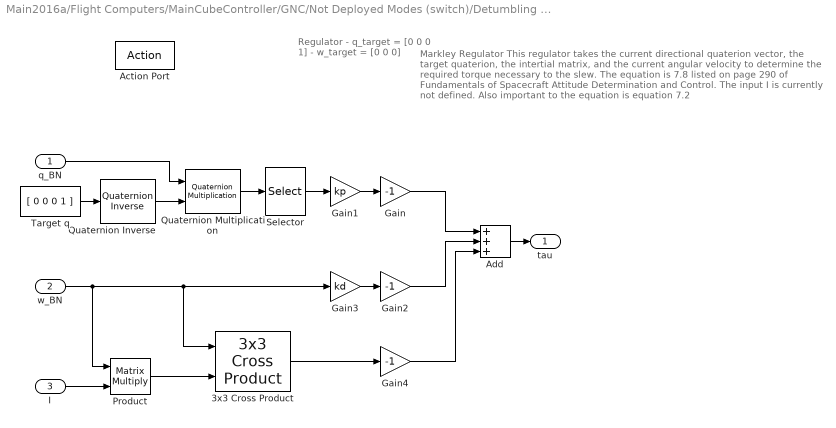
== system Main2016a/Flight Computers/MainCubeController/GNC/Not Deployed Modes (switch)/Detumbling Slew ==
  note: Regulator
      | - q_target = [0 0 0 1]
      | - w_target = [0 0 0]
  note: Markley Regulator
      | This regulator takes the current directional quaterion vector, the target quaterion, the intertial matrix, and the current angular velocity to determine the required torque necessary to the slew.
      |
      | The equation is 7.8 listed on page 290 of Fundamentals of Spacecraft Attitude Determination and Control. The input I is currently not defined. Also important to the equation is equation 7.2
  q_BN : Inport
  w_BN : Inport  Port=2
  "I " : Inport  Port=3
  Action Port : ActionPort
  3x3 Cross Product : aerolibutil/3x3 Cross Product
  Add : Sum  Inputs=+++
  Gain : Gain  Gain=-1
  Gain1 : Gain  Gain=kp
  Gain2 : Gain  Gain=-1
  Gain3 : Gain  Gain=kd
  Gain4 : Gain  Gain=-1
  Product : Product  Multiplication=Matrix(*)
  Quaternion Inverse : aerolibutil/Quaternion Inverse
  Quaternion Multiplication : aerolibutil/Quaternion Multiplication
  Selector : Selector  InputPortWidth=4  IndexOptions=Index vector (dialog)  Indices=[1 2 3]  OutputSizes=1
  Target q : Constant  Value=[ 0 0 0 1 ]
  tau : Outport
  wires:
  q_BN/1 -> Quaternion Multiplication/1
  Quaternion Inverse/1 -> Quaternion Multiplication/2
  Target q/1 -> Quaternion Inverse/1
  Quaternion Multiplication/1 -> Selector/1
  Selector/1 -> Gain1/1
  Gain1/1 -> Gain/1
  Gain3/1 -> Gain2/1
  w_BN/1 -> Product/1, 3x3 Cross Product/1, Gain3/1
  Add/1 -> tau/1
  Gain/1 -> Add/1
  Gain2/1 -> Add/2
  "I "/1 -> Product/2
  Product/1 -> 3x3 Cross Product/2
  3x3 Cross Product/1 -> Gain4/1
  Gain4/1 -> Add/3

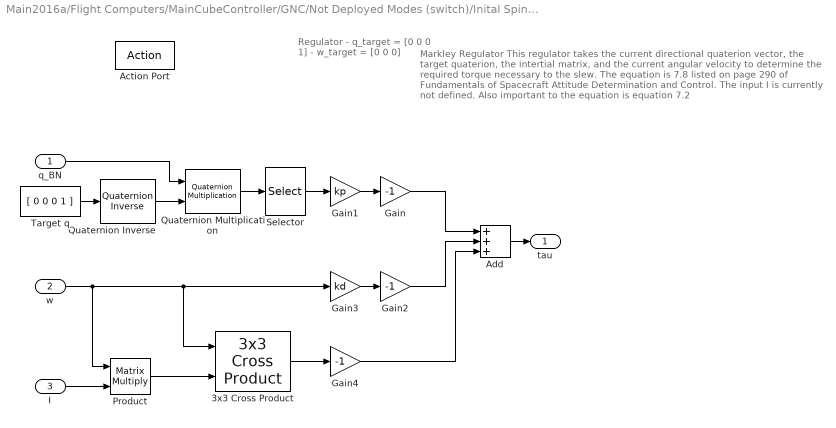
== system Main2016a/Flight Computers/MainCubeController/GNC/Not Deployed Modes (switch)/Inital Spin Up ==
  note: Regulator
      | - q_target = [0 0 0 1]
      | - w_target = [0 0 0]
  note: Markley Regulator
      | This regulator takes the current directional quaterion vector, the target quaterion, the intertial matrix, and the current angular velocity to determine the required torque necessary to the slew.
      |
      | The equation is 7.8 listed on page 290 of Fundamentals of Spacecraft Attitude Determination and Control. The input I is currently not defined. Also important to the equation is equation 7.2
  q_BN : Inport
  w : Inport  Port=2
  "I " : Inport  Port=3
  Action Port : ActionPort  ActionType=case
  3x3 Cross Product : aerolibutil/3x3 Cross Product
  Add : Sum  Inputs=+++
  Gain : Gain  Gain=-1
  Gain1 : Gain  Gain=kp
  Gain2 : Gain  Gain=-1
  Gain3 : Gain  Gain=kd
  Gain4 : Gain  Gain=-1
  Product : Product  Multiplication=Matrix(*)
  Quaternion Inverse : aerolibutil/Quaternion Inverse
  Quaternion Multiplication : aerolibutil/Quaternion Multiplication
  Selector : Selector  InputPortWidth=4  IndexOptions=Index vector (dialog)  Indices=[1 2 3]  OutputSizes=1
  Target q : Constant  Value=[ 0 0 0 1 ]
  tau : Outport
  wires:
  q_BN/1 -> Quaternion Multiplication/1
  Quaternion Inverse/1 -> Quaternion Multiplication/2
  Target q/1 -> Quaternion Inverse/1
  Quaternion Multiplication/1 -> Selector/1
  Selector/1 -> Gain1/1
  Gain1/1 -> Gain/1
  Gain3/1 -> Gain2/1
  w/1 -> Product/1, 3x3 Cross Product/1, Gain3/1
  Add/1 -> tau/1
  Gain/1 -> Add/1
  Gain2/1 -> Add/2
  "I "/1 -> Product/2
  Product/1 -> 3x3 Cross Product/2
  3x3 Cross Product/1 -> Gain4/1
  Gain4/1 -> Add/3

== system Main2016a/Flight Computers/MainCubeController/GNC/Not Deployed Modes (switch)/Null Case1 ==
  Action Port : ActionPort
  Constant : Constant  Value=[ 0 0 0 ]
  Out1 : Outport
  wires:
  Constant/1 -> Out1/1

== system Main2016a/Flight Computers/MainCubeController/GNC/Not Deployed Modes (switch)/Seek EKF Convergence ==
  Action Port : ActionPort  ActionType=case
  Constant : Constant  Value=[ 0 0 0 ]
  Out1 : Outport
  wires:
  Constant/1 -> Out1/1

== system Main2016a/Flight Computers/MainCubeController/GNC/Not Deployed Modes (switch)/Sun Pointing ==
  note: Regulator
      | - q_target = [0 0 1 0]
      | - w_target = [0 0 0]
  q : Inport
  w_BN : Inport  Port=2
  Action Port : ActionPort
  Add : Sum
  Add1 : Sum  Inputs=+-
  Gain : Gain  Gain=-1
  Gain1 : Gain  Gain=kp
  Gain2 : Gain  Gain=-1
  Gain3 : Gain  Gain=kd
  Quaternion Inverse : aerolibutil/Quaternion Inverse
  Quaternion Multiplication : aerolibutil/Quaternion Multiplication
  Selector : Selector  InputPortWidth=4  IndexOptions=Index vector (dialog)  Indices=[1 2 3]  OutputSizes=1
  Target q : Constant  Value=[ 0 0 1 0 ]
  Target w : Constant  Value=[ 0 0 0 ]
  tau : Outport
  wires:
  q/1 -> Quaternion Multiplication/1
  Quaternion Inverse/1 -> Quaternion Multiplication/2
  Target q/1 -> Quaternion Inverse/1
  Quaternion Multiplication/1 -> Selector/1
  Selector/1 -> Gain1/1
  Gain1/1 -> Gain/1
  Gain3/1 -> Gain2/1
  w_BN/1 -> Add1/1
  Add/1 -> tau/1
  Gain/1 -> Add/1
  Gain2/1 -> Add/2
  Target w/1 -> Add1/2
  Add1/1 -> Gain3/1

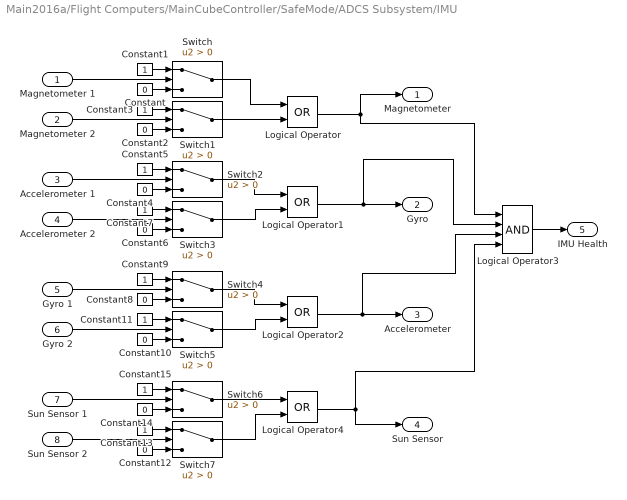
== system Main2016a/Flight Computers/MainCubeController/SafeMode/ADCS Subsystem/IMU ==
  Magnetometer 1 : Inport
  Magnetometer 2 : Inport  Port=2
  Accelerometer 1 : Inport  Port=3
  " Accelerometer 2" : Inport  Port=4
  Gyro 1 : Inport  Port=5
  Gyro 2 : Inport  Port=6
  Sun Sensor 1 : Inport  Port=7
  Sun Sensor 2 : Inport  Port=8
  Constant{,2,4,6,8,10,12,14} (8 alike) : Constant  Value=0
  Constant{1,3,5,7,9,11,13,15} (8 alike) : Constant
  Logical Operator{,1..2,4} (4 alike) : Logic  Operator=OR  AllPortsSameDT=off  OutDataTypeStr=boolean
  Logical Operator3 : Logic  Inputs=4  AllPortsSameDT=off  OutDataTypeStr=boolean
  Switch{,1..7} (8 alike) : Switch  Criteria=u2 > Threshold
  Magnetometer : Outport
  "Gyro " : Outport  Port=2
  Accelerometer : Outport  Port=3
  "Sun Sensor " : Outport  Port=4
  IMU Health : Outport  Port=5
  wires:
  Logical Operator3/1 -> IMU Health/1
  Switch7/1 -> Logical Operator4/2
  Constant12/1 -> Switch7/3
  Constant13/1 -> Switch7/1
  Switch6/1 -> Logical Operator4/1
  Constant14/1 -> Switch6/3
  Constant15/1 -> Switch6/1
  Logical Operator4/1 -> Logical Operator3/4, "Sun Sensor "/1
  Switch5/1 -> Logical Operator2/2
  Constant10/1 -> Switch5/3
  Constant11/1 -> Switch5/1
  Switch4/1 -> Logical Operator2/1
  Constant8/1 -> Switch4/3
  Constant9/1 -> Switch4/1
  Switch3/1 -> Logical Operator1/2
  Constant6/1 -> Switch3/3
  Constant7/1 -> Switch3/1
  Switch2/1 -> Logical Operator1/1
  Constant4/1 -> Switch2/3
  Constant5/1 -> Switch2/1
  Switch1/1 -> Logical Operator/2
  Constant2/1 -> Switch1/3
  Constant3/1 -> Switch1/1
  Switch/1 -> Logical Operator/1
  Constant/1 -> Switch/3
  Constant1/1 -> Switch/1
  Magnetometer 1/1 -> Switch/2
  Logical Operator2/1 -> Accelerometer/1, Logical Operator3/3
  Logical Operator1/1 -> "Gyro "/1, Logical Operator3/2
  Logical Operator/1 -> Logical Operator3/1, Magnetometer/1
  Magnetometer 2/1 -> Switch1/2
  Gyro 1/1 -> Switch4/2
  Gyro 2/1 -> Switch5/2
  Sun Sensor 1/1 -> Switch6/2
  Sun Sensor 2/1 -> Switch7/2
  " Accelerometer 2"/1 -> Switch3/2
  Accelerometer 1/1 -> Switch2/2

== system Main2016a/Flight Computers/MainCubeController/SafeMode/ADCS Subsystem/Magnetic Torquers ==
  Magnetorquer X1 : Inport
  Magnetometer Y1 : Inport  Port=2
  Magnetometer Z1 : Inport  Port=3
  Constant : Constant  Value=0
  Constant1 : Constant
  Constant4 : Constant  Value=0
  Constant5 : Constant
  Constant8 : Constant  Value=0
  Constant9 : Constant
  Logical Operator3 : Logic  Inputs=3  AllPortsSameDT=off  OutDataTypeStr=boolean
  Switch : Switch  Criteria=u2 > Threshold
  Switch2 : Switch  Criteria=u2 > Threshold
  Switch4 : Switch  Criteria=u2 > Threshold
  X Torquer Status : Outport
  "Y Torquer Status " : Outport  Port=2
  Z Torquer Status : Outport  Port=3
  Actuator Health : Outport  Port=4
  wires:
  Logical Operator3/1 -> Actuator Health/1
  Constant8/1 -> Switch4/3
  Constant9/1 -> Switch4/1
  Magnetometer Z1/1 -> Switch4/2
  Constant4/1 -> Switch2/3
  Constant5/1 -> Switch2/1
  Magnetometer Y1/1 -> Switch2/2
  Constant/1 -> Switch/3
  Constant1/1 -> Switch/1
  Magnetorquer X1/1 -> Switch/2
  Switch4/1 -> Z Torquer Status/1, Logical Operator3/3
  Switch2/1 -> "Y Torquer Status "/1, Logical Operator3/2
  Switch/1 -> X Torquer Status/1, Logical Operator3/1

== matlab function Main2016a/Dynamics/Rigid Dynamics/MATLAB Function ==
  data: burn input; u1 output; solardeploy input
function u1 = fcn(burn,solardeploy)
%#codegen

u1 = burn;

end

== matlab function Main2016a/Inputs/Choose Mode ==
  data: time input; OM output; OpTimes input; OpModes input; SeperationTime input; SEPC output; SDC output; SolarDeployTime input
function [OM , SEPC , SDC] = ...
    ModeSwitching(time,OpTimes,OpModes,SeperationTime,SolarDeployTime)
%#codegen

tind = find(time > OpTimes);

if isempty(tind)
    i = 1;
else
    i = tind(end);
end

OM = OpModes(i);

if time > SeperationTime
    SEPC = 1;
else
    SEPC = 0;
end

if time > SolarDeployTime
    SDC = 1;
else
    SDC = 0;
end

end

== matlab function Main2016a/Flight Computers/MainCubeController/SafeMode/ACS State Machine Mode determination ==
  data: SafeMode_In input; SafeMode_Out output; SafedOpMode output; PwbMEX output; x input; t input; ADCSs input; EKFAE input; EKFhs input; OpMode input; PbOpMode input; SeperationCommand input; xold input; xnew output
function [SafeMode_Out, SafedOpMode, PwbMEX, xnew] = fcn(SafeMode_In, x, ...
    t, ADCSs, EKFAE, EKFhs, OpMode, PbOpMode, SeperationCommand, xold)
%#codegen
% x = t, ADCSs, EKFAE, EKFhs, OpMode, PbOpMode, SeperationCommand;
%% States of State Machine
% Time (From Deployment)​           t
% ADCS Health Status​               ADCSs
% EKF Attitude Estimate​            EKFAE
% EKF Health Status​                EKFhs
% Current Status                   OpMode
% PowerBoard Override              PbOpMode
% Deployed or not                  SeperationCommand

%% ADCSs
% ADCS Functional Status            ADCS_Fs
% ADCS Sectional Status             ADCS_Ss
% ADCS Component Status             ADCS_Cs

%%%%%%%%%%%%%%%%%%%%%%%%%%% MODE FLAGS %%%%%%%%%%%%%%%%%%%%%%%%%%%%%%%%%%%%
% 1 = Initial Charging Mode
% 2 = System Verification and Check Mode
% 3 = EPS THS Ping Mode
% 4 = FC THS Ping Mode
% 5 = Detumble Mode
% 6 = Sun Pointing Mode
% 7 = Spin Up Mode
% 8 = End Satellite Deployment Mode
% 9 = Normal OPS Mode
% 10 = Eclipse/Sleep Mode Mode
% 11 = Safe State Mode
% 12 = SeekingEKFConvergence

%% PwbMEX 
% PwbMEX is the error signal sent to the PowerBoard containing important
% information about the status of the ADCSs components as seen in safe
% mode. Informs that Safe Mode was entered, and requests an exit, as well
% as informs of the subsystem components that were not functionoing
% properly.
% MORE INFORMATION TO BE PROVIDED AFTER DISCUSSION WITH PADRAIG ON FORMAT
% AND NEED
PwbMEX = [0];
% Niccolo Porcari 2017

%%%%%%%%%%%%%%%%%%%%%%%%%%%%%%%%%%%%%%%%%%%%%%%%%%%%%%%%%%%%%%%%%%%%%%%%%%%

    if x.t > 2700 % seconds
        %% INITIAL CHECKS (check if in SafeMode)
        if (SafeMode_In == true || x.PbOpMode == 11)
            PwbMEX = [1];
            % FIND A WAY TO INFORM POWERBOARD
            if (x.PbOpMode ~= 11)
                SafeMode_In = false;
                PwbMEX = [0]; % reset error message to powerboard
                x.OpMode = x.PbOMode;
            else
                x.OpMode = 11;
                %% SAFE MODE OCCURS
                errorPositions = findADCSfault(ADCSs);
                % INFORM POWERBOARD Of location of error
                PwbMEX = [PwbMEX errorPositions]; %%% PARTIAL ONLY
            end
        else
            %% SECTION for all modes where  ADCS is operational 
            % Pretend EKFhs is a boolean for now:
            if (x.OpMode == 5) || (x.OpMode == 6) || (x.OpMode == 7) || (x.OpMode == 9) || (x.OpMode == 10)
                if x.ADCSs(1) == false % Failure of ADCS trips Safe State Mode
                    x.OpMode = 11;
                    PwbMEX = [1];
                    SafeMode_in = true;
                elseif EKFhs ~= true % Check validity of EKF estimate
                    x.OpMode = 12;  % Need to think of what we're gonna do if 
                                    % the EKF isn't technically accurate yet
                elseif EKFhs == true
                    x.OpMode = x.PbOpMode;
                end
            end
        end
        
        %% RESET OpMode to match PbOpMode 
        if (x.PbOpMode ~= x.OpMode && x.OpMode ~= 12) % set mode to match powerboard demand
            x.OpMode = x.PbOpMode;
        end
        xnew = x;
    end
end

== matlab function Main2016a/PowerBoard Simulation/Choose Mode ==
  data: PwbMEX input; time input; OM output; OpTimes input; OpModes input; SeperationTime input; SEPC output; SDC output; SolarDeployTime input
function [OM , SEPC , SDC] = ...
    ModeSwitching(PwbMEX, time,OpTimes,OpModes,SeperationTime,SolarDeployTime)
%#codegen

tind = find(time > OpTimes);

if isempty(tind)
    i = 1;
else
    i = tind(end);
end

OM = OpModes(i);

if time > SeperationTime
    SEPC = 1;
else
    SEPC = 0;
end

if time > SolarDeployTime
    SDC = 1;
else
    SDC = 0;
end

end

== matlab function Main2016a/Flight Computers/MainCubeController/Navigation/Torque Coil Management/B_Q_N ==
  data: q_BN input; DCM output
function DCM = fcn(q_BN)
	DCM = q2dcm(q_BN);
end
